simulink model "fuzzywork"  (Simulink 5.0)
settings: Solver=ode1  StartTime=0.0  StopTime=70.0  RelTol=1e-3
PreLoadFcn:
  | new=readfis('new')
libraries: pci1711 x3, fuzblock x2
settings Model: LastModifiedBy=AD  SimulationMode=external  BooleanDataType=off  RTWOptions="-aEnforceIntegerDowncast=1 -aExtMode=0 -aExtModeTesting=0 -aFoldNonRolledExpr=1 -aForceParamTrailComments=0 -aGenerateComments=1 -aGenerateReport=0 -aIgnoreCustomStorageClasses=1 -aIncDataTypeInIds=0 -aIncHierarchyInIds=0 -aInlineInvariantSignals=0 -aInlineParameters=0 -aInlinedPrmAccess=\"Literals\" -aLocalBlockOutputs=1 -aLogVarNameModifier=\"rt_\" -aMaxRTWIdLen=31 -aPrefixModelToSubsysFcnNames=1 -aRTWVerbose=1 -aRollThreshold=5 -aShowEliminatedStatements=0"

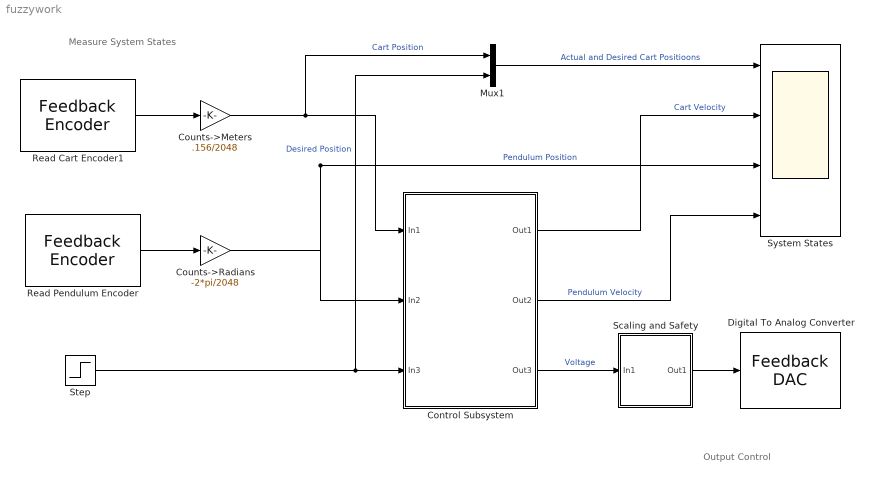
== system fuzzywork ==
  note: Measure System States
  note: Output Control
  Control Subsystem : Subsystem
  Counts->Meters : Gain  Gain=.156/2048  SaturateOnIntegerOverflow=on
  Counts->Radians : Gain  Gain=-2*pi/2048  SaturateOnIntegerOverflow=on
  Digital To Analog Converter : pci1711/Advantech  PCI1711 I//O Board Lib/Feedback DAC  channel=0  range=0  tsamp=0.001  hwAccess=on
  Mux1 : Mux  Inputs=2
  Read Cart Encoder1 : pci1711/Advantech  PCI1711 I//O Board Lib/Feedback Encoder   channel=0  offset=0  tsamp=0.001  hwAccess=on
  Read Pendulum Encoder : pci1711/Advantech  PCI1711 I//O Board Lib/Feedback Encoder   channel=1  offset=-1024  tsamp=0.001  hwAccess=on
  Scaling and Safety : Subsystem
  Step : Step  SampleTime=0
  System States : Scope  NumInputPorts=4
      settings: TimeRange=70  YMin=-0.5~-1~-6~-15  YMax=0.5~1~6~15  Decimation=0.1  SampleInput=on  SampleTime=0.01
  wires:
  Counts->Meters/1 -> Control Subsystem/1(In1), Mux1/1  "Cart Position"
  Counts->Radians/1 -> Control Subsystem/2(In2), System States/3  "Pendulum Position"
  Scaling and Safety/1(Out1) -> Digital To Analog Converter/1
  Step/1 -> Control Subsystem/3(In3), Mux1/2  "Desired Position"
  Control Subsystem/3(Out3) -> Scaling and Safety/1(In1)  "Voltage"
  Mux1/1 -> System States/1  "Actual and Desired Cart Positioons"
  Read Cart Encoder1/1 -> Counts->Meters/1
  Read Pendulum Encoder/1 -> Counts->Radians/1
  Control Subsystem/1(Out1) -> System States/2  "Cart Velocity"
  Control Subsystem/2(Out2) -> System States/4  "Pendulum Velocity"

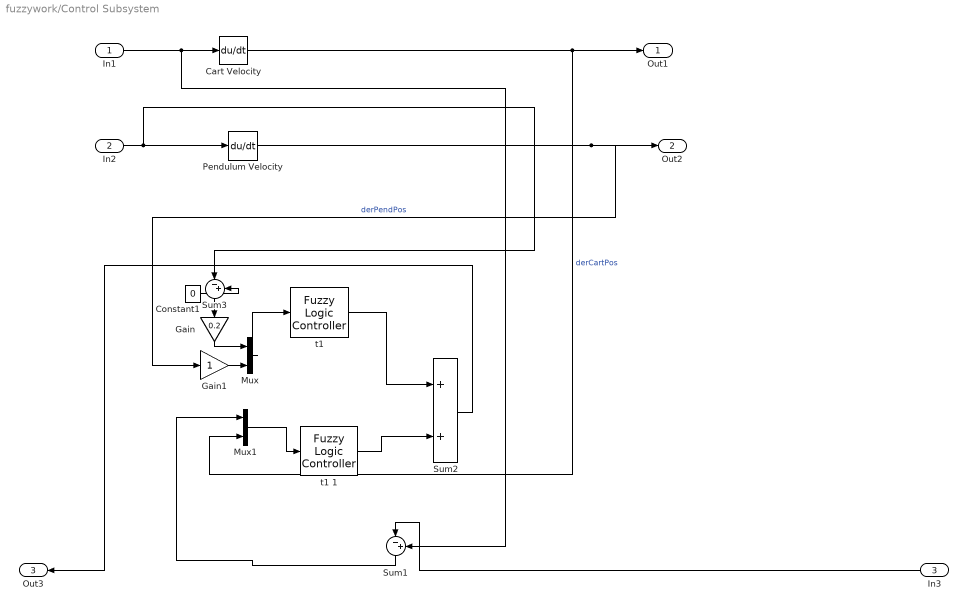
== system fuzzywork/Control Subsystem ==
  In1 : Inport
  In2 : Inport  Port=2
  In3 : Inport  Orientation=left  Port=3
  Cart Velocity : Derivative
  Constant1 : Constant  Value=0
  Gain : Gain  Orientation=down  Gain=0.2  SaturateOnIntegerOverflow=on
  Gain1 : Gain  SaturateOnIntegerOverflow=on
  Mux : Mux  Inputs=2
  Mux1 : Mux  Inputs=2
  Pendulum Velocity : Derivative
  Sum1 : Sum  Orientation=down  Inputs=|-+  SaturateOnIntegerOverflow=on
  Sum2 : Sum  SaturateOnIntegerOverflow=on
  Sum3 : Sum  Orientation=down  Inputs=|-+  SaturateOnIntegerOverflow=on
  "t1 " : fuzblock/Fuzzy Logic  Controller  fis=new
  t1 1 : fuzblock/Fuzzy Logic  Controller  fis=new
  Out1 : Outport
  Out2 : Outport  Port=2
  Out3 : Outport  Orientation=left  Port=3
  wires:
  In3/1 -> Sum1/1
  In2/1 -> Pendulum Velocity/1, Sum3/1
  In1/1 -> Cart Velocity/1, Sum1/2
  Pendulum Velocity/1 -> Out2/1, Gain1/1  "derPendPos"
  Cart Velocity/1 -> Out1/1, Mux1/2  "derCartPos"
  t1 1/1 -> Sum2/2
  Gain/1 -> Mux/1
  Gain1/1 -> Mux/2
  "t1 "/1 -> Sum2/1
  Sum3/1 -> Gain/1
  Constant1/1 -> Sum3/2
  Mux/1 -> "t1 "/1
  Sum1/1 -> Mux1/1
  Mux1/1 -> t1 1/1
  Sum2/1 -> Out3/1

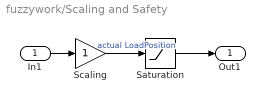
== system fuzzywork/Scaling and Safety ==
  In1 : Inport
  Saturation : Saturate  UpperLimit=2.5  LowerLimit=-2.5
  Scaling : Gain  SaturateOnIntegerOverflow=on
  Out1 : Outport
  wires:
  Scaling/1 -> Saturation/1  "actual LoadPosition"
  In1/1 -> Scaling/1
  Saturation/1 -> Out1/1
